simulink model "FullSystemSim_old"  (R2020a)
settings: Solver=VariableStepAuto  StartTime=0.0  StopTime=T_sim  RelTol=1e-3
values from neighbouring files (symbols this model uses):
  a_friction = 0    [FullSystem.m]
  b_friction = 1.19    [FullSystem.m]
  C_T_matrix = ex2(2:12,2:21)'    [FullSystem.m]
  J_wind = 5.245e-6 * 1000    (= 0.005245)    [FullSystem.m]
  K_t = 0.023    [FullSystem.m]    (also in WindTurbine.m = 82.8991502528)
  K_v = 0.023 / pi * 30    (= 0.219633821467)    [FullSystem.m]    (also in WindTurbine.m = 115.191730632)
  lambda_data_x = ex1(6, :)'    [FullSystem.m]
  lambda_opt = 2.1    [FullSystem.m]
  omega_0 = 100    [FullSystem.m]    (also in SystemControl_script.m = 100:)
  P_max_EL = 3    [FullSystem.m]
  P_max_FC = 1    [FullSystem.m]
  P_max_LED = 12*0.16*4    (= 7.68)    [FullSystem.m]
  P_max_SP = 0.5    [FullSystem.m]
  P_max_WT = 0.2    [FullSystem.m]
  R_LED_max = 75/4    (= 18.75)    [FullSystem.m]
  R_motor = 22.222    [FullSystem.m]
  R_turbine = 0.15    [FullSystem.m]    (also in SystemControl_script.m)
  r_wind_data_x = ex1(7, :)'    [FullSystem.m]
  rho_air = 1.225    [FullSystem.m]
  step_size = T_sim/n    (= 0.04)    [FullSystem.m]
  V_w_data_x = ex1(8,:)'    [FullSystem.m]
undefined symbols (not defined in the file or in its folder): DiscIntNeverNeededParam
libraries: fl_lib x37, nesl_utility x26, ee_lib x19, eePwmGenerator x4, simulink x2
settings Model: Creator=thequ  LastModifiedBy=fabia
settings DebuggingCC: ArithmeticOperatorsInVariantConditions=warning
settings SFSimCC: CustomCodeUndefinedFunction=UseInterfaceOnly

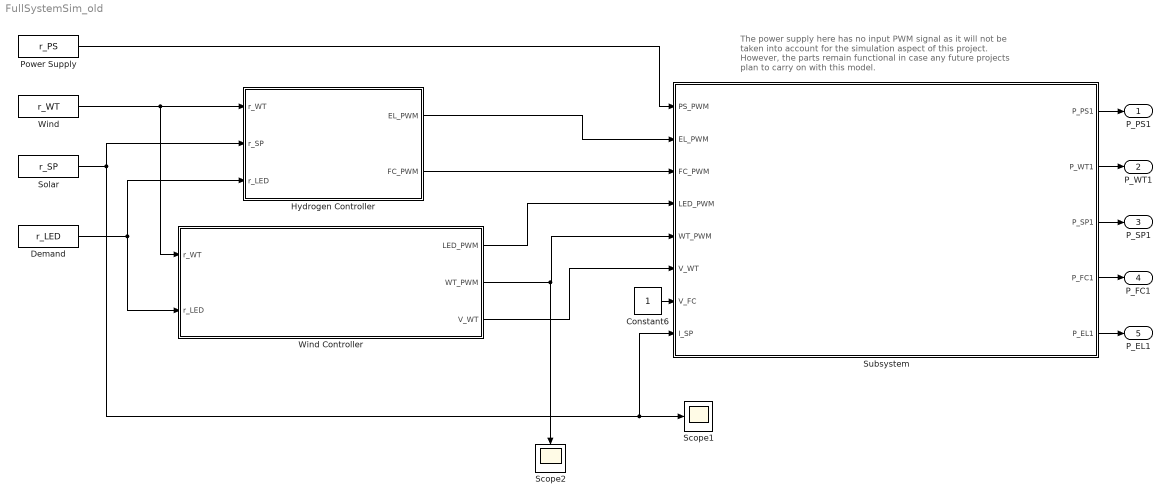
== system FullSystemSim_old ==
  note: The power supply here has no input PWM signal as it will not
      | be taken into account for the simulation aspect of this project.
      | However, the parts remain functional in case any future
      | projects plan to carry on with this model.
  Constant6 : Constant
  Demand : FromWorkspace  VariableName=r_LED  SampleTime=step_size  Interpolate=off  OutputAfterFinalValue=Holding final value
  Hydrogen Controller : Subsystem
  Power Supply : FromWorkspace  VariableName=r_PS  SampleTime=step_size  Interpolate=off  OutputAfterFinalValue=Holding final value
  Scope1 : Scope
  Scope2 : Scope
  Solar : FromWorkspace  VariableName=r_SP  SampleTime=step_size  Interpolate=off  OutputAfterFinalValue=Holding final value
  Subsystem : Subsystem
  Wind : FromWorkspace  VariableName=r_WT  SampleTime=step_size  Interpolate=off  OutputAfterFinalValue=Holding final value
  Wind Controller : Subsystem
  P_PS1 : Outport
  P_WT1 : Outport  Port=2
  P_SP1 : Outport  Port=3
  P_FC1 : Outport  Port=4
  P_EL1 : Outport  Port=5
  wires:
  Power Supply/1 -> Subsystem/1(PS_PWM)
  Subsystem/1(P_PS1) -> P_PS1/1
  Subsystem/2(P_WT1) -> P_WT1/1
  Subsystem/3(P_SP1) -> P_SP1/1
  Subsystem/4(P_FC1) -> P_FC1/1
  Subsystem/5(P_EL1) -> P_EL1/1
  Demand/1 -> Hydrogen Controller/3(r_LED), Wind Controller/2(r_LED)
  Wind Controller/3(V_WT) -> Subsystem/6(V_WT)
  Constant6/1 -> Subsystem/7(V_FC)
  Wind/1 -> Wind Controller/1(r_WT), Hydrogen Controller/1(r_WT)
  Solar/1 -> Hydrogen Controller/2(r_SP), Subsystem/8(I_SP), Scope1/1
  Wind Controller/2(WT_PWM) -> Subsystem/5(WT_PWM), Scope2/1
  Wind Controller/1(LED_PWM) -> Subsystem/4(LED_PWM)
  Hydrogen Controller/1(EL_PWM) -> Subsystem/2(EL_PWM)
  Hydrogen Controller/2(FC_PWM) -> Subsystem/3(FC_PWM)

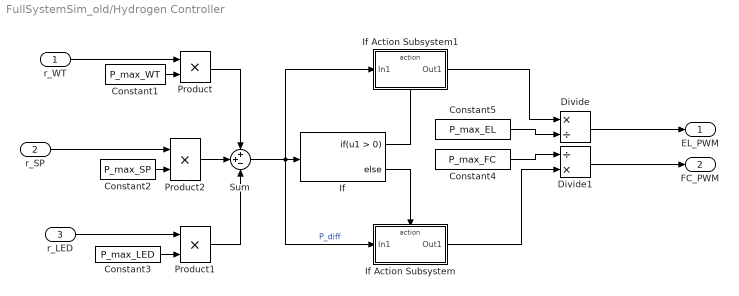
== system FullSystemSim_old/Hydrogen Controller ==
  r_WT : Inport
  r_SP : Inport  Port=2
  r_LED : Inport  Port=3
  Constant1 : Constant  Value=P_max_WT
  Constant2 : Constant  Value=P_max_SP
  Constant3 : Constant  Value=P_max_LED
  Constant4 : Constant  Value=P_max_FC
  Constant5 : Constant  Value=P_max_EL
  Divide : Product  Inputs=*/
  Divide1 : Product  Inputs=/*
  If : If
  If Action Subsystem : Subsystem  TreatAsAtomicUnit=on
  If Action Subsystem1 : Subsystem  TreatAsAtomicUnit=on
  Product : Product
  Product1 : Product
  Product2 : Product
  Sum : Sum  Inputs=++-
  EL_PWM : Outport
  FC_PWM : Outport  Port=2
  wires:
  Divide1/1 -> FC_PWM/1
  Product/1 -> Sum/1
  Divide/1 -> EL_PWM/1
  r_WT/1 -> Product/1
  If Action Subsystem/1(Out1) -> Divide1/2
  Constant5/1 -> Divide/2
  If/2 -> If Action Subsystem/Action
  Product1/1 -> Sum/3
  Sum/1 -> If Action Subsystem1/1(In1), If Action Subsystem/1(In1), If/1  "P_diff"
  Constant1/1 -> Product/2
  Constant4/1 -> Divide1/1
  If/1 -> If Action Subsystem1/Action
  If Action Subsystem1/1(Out1) -> Divide/1
  Constant3/1 -> Product1/2
  Constant2/1 -> Product2/2
  Product2/1 -> Sum/2
  r_LED/1 -> Product1/1
  r_SP/1 -> Product2/1

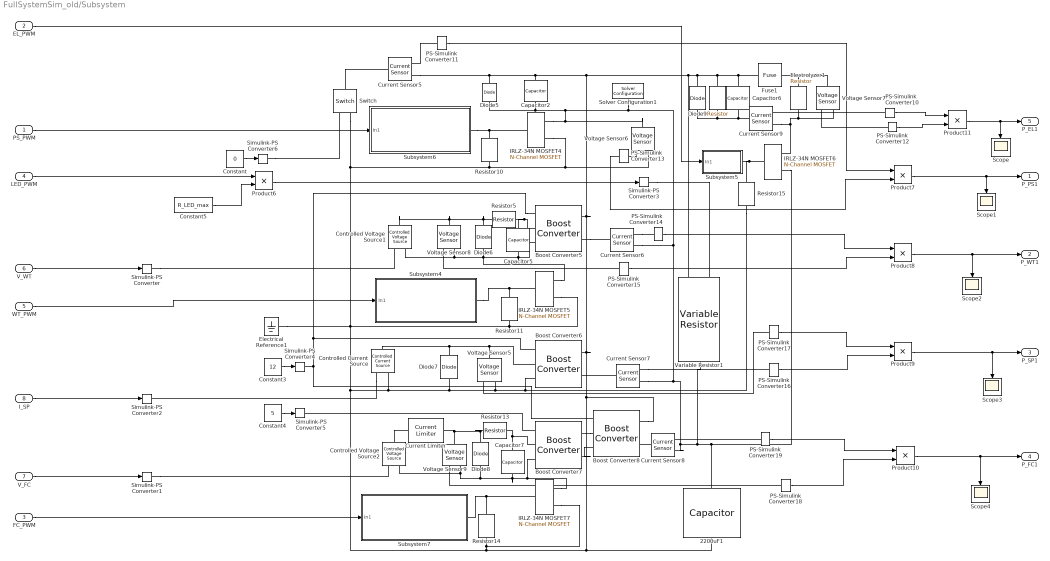
== system FullSystemSim_old/Subsystem ==
  PS_PWM : Inport
  EL_PWM : Inport  Port=2
  FC_PWM : Inport  Port=3
  LED_PWM : Inport  Port=4
  WT_PWM : Inport  Port=5
  V_WT : Inport  Port=6
  V_FC : Inport  Port=7
  I_SP : Inport  Port=8
  " " : fl_lib/Electrical/Electrical Elements/Resistor  R=16 Ohm  i_specify=off  i_priority=None  i=0 A  i_nominal_specify=off  i_nominal_unit=A  i_nominal_value=1  v_specify=off  v_priority=None  v=0 V  v_nominal_specify=off  v_nominal_unit=V  v_nominal_value=1
  2200uF1 : fl_lib/Electrical/Electrical Elements/Capacitor  c=2200 uF  r=0.014 Ohm  g=0 1/Ohm  i_specify=off  i_priority=None  i=0 A  i_nominal_specify=off  i_nominal_unit=A  i_nominal_value=1  v_specify=off  v_priority=None  v=0 V  v_nominal_specify=off  v_nominal_unit=V  v_nominal_value=1  vc_specify=off  vc_priority=High  vc=0 V  vc_nominal_specify=off  vc_nominal_unit=V  vc_nominal_value=1
  Boost Converter5 : ee_lib/Semiconductors & Converters/Converters/Boost Converter  device_type=4  Vf=0.8 V  Ron=0.001 Ohm  Rds=0.08 Ohm  Goff=1e-5 1/Ohm  Vth=2 V  Vgt=1 V  Vgt_off=-1 V  Ih=1 A  diode_param=2  diode_Vf=0.8 V  diode_Ron=0.001 Ohm  diode_Goff=1e-5 1/Ohm  diode_C=50 nF  diode_iRM=-235 A  diode_iF=300 A  diode_idot=-50 A/us  diode_trr_param=1  diode_trr_factor=3  diode_trr=15 us  diode_Qrr=1500 s*uA  Lf=1e-6 H  Cf=1e-7 F  Rf=1e-6 Ohm  snubber_type=0  Rs=0.1 Ohm  Cs=1e-7 F
      settings: SourceProductBaseCode=PS  InternalSimscapePortConfiguration="{\"Bottom\":[],\"Left\":[{\"id\":\"G\",\"label\":\"G\",\"type\":\"input\"},{\"id\":\"p1\",\"label\":\"1+\",\"type\":\"foundation.electrical.electrical\"},{\"id\":\"n1\",\"label\":\"1-\",\"type\":\"foundation.electrical.electrical\"}],\"Right\":[{\"id\":\"p2\",\"label\":\"2+\",\"type\":\"foundation.electrical.electrical\"},{\"id\":\"n2\",\"label\":\"2-\",\"type\":\"foundation.electrical.electrical\"}],\"Top\":[]}"
  Boost Converter6 : ee_lib/Semiconductors & Converters/Converters/Boost Converter  device_type=4  Vf=0.8 V  Ron=0.001 Ohm  Rds=0.08 Ohm  Goff=1e-5 1/Ohm  Vth=2 V  Vgt=1 V  Vgt_off=-1 V  Ih=1 A  diode_param=2  diode_Vf=0.8 V  diode_Ron=0.001 Ohm  diode_Goff=1e-5 1/Ohm  diode_C=50 nF  diode_iRM=-235 A  diode_iF=300 A  diode_idot=-50 A/us  diode_trr_param=1  diode_trr_factor=3  diode_trr=15 us  diode_Qrr=1500 s*uA  Lf=1e-6 H  Cf=1e-7 F  Rf=1e-6 Ohm  snubber_type=0  Rs=0.1 Ohm  Cs=1e-7 F
      settings: SourceProductBaseCode=PS  InternalSimscapePortConfiguration="{\"Bottom\":[],\"Left\":[{\"id\":\"G\",\"label\":\"G\",\"type\":\"input\"},{\"id\":\"p1\",\"label\":\"1+\",\"type\":\"foundation.electrical.electrical\"},{\"id\":\"n1\",\"label\":\"1-\",\"type\":\"foundation.electrical.electrical\"}],\"Right\":[{\"id\":\"p2\",\"label\":\"2+\",\"type\":\"foundation.electrical.electrical\"},{\"id\":\"n2\",\"label\":\"2-\",\"type\":\"foundation.electrical.electrical\"}],\"Top\":[]}"
  Boost Converter7 : ee_lib/Semiconductors & Converters/Converters/Boost Converter  device_type=4  Vf=0.8 V  Ron=0.001 Ohm  Rds=0.080 Ohm  Goff=1e-5 1/Ohm  Vth=0.9 V  Vgt=1 V  Vgt_off=-1 V  Ih=1 A  diode_param=2  diode_Vf=0.8 V  diode_Ron=0.001 Ohm  diode_Goff=1e-5 1/Ohm  diode_C=50 nF  diode_iRM=-235 A  diode_iF=300 A  diode_idot=-50 A/us  diode_trr_param=1  diode_trr_factor=3  diode_trr=15 us  diode_Qrr=1500 s*uA  Lf=1e-6 H  Cf=1e-7 F  Rf=1e-6 Ohm  snubber_type=0  Rs=0.1 Ohm  Cs=1e-7 F
      settings: SourceProductBaseCode=PS  InternalSimscapePortConfiguration="{\"Bottom\":[],\"Left\":[{\"id\":\"G\",\"label\":\"G\",\"type\":\"input\"},{\"id\":\"p1\",\"label\":\"1+\",\"type\":\"foundation.electrical.electrical\"},{\"id\":\"n1\",\"label\":\"1-\",\"type\":\"foundation.electrical.electrical\"}],\"Right\":[{\"id\":\"p2\",\"label\":\"2+\",\"type\":\"foundation.electrical.electrical\"},{\"id\":\"n2\",\"label\":\"2-\",\"type\":\"foundation.electrical.electrical\"}],\"Top\":[]}"
  Boost Converter8 : ee_lib/Semiconductors & Converters/Converters/Boost Converter  device_type=4  Vf=0.8 V  Ron=0.001 Ohm  Rds=0.08 Ohm  Goff=1e-5 1/Ohm  Vth=2 V  Vgt=1 V  Vgt_off=-1 V  Ih=1 A  diode_param=2  diode_Vf=0.8 V  diode_Ron=0.001 Ohm  diode_Goff=1e-5 1/Ohm  diode_C=50 nF  diode_iRM=-235 A  diode_iF=300 A  diode_idot=-50 A/us  diode_trr_param=1  diode_trr_factor=3  diode_trr=15 us  diode_Qrr=1500 s*uA  Lf=1e-6 H  Cf=1e-7 F  Rf=1e-6 Ohm  snubber_type=0  Rs=0.1 Ohm  Cs=1e-7 F
      settings: SourceProductBaseCode=PS  InternalSimscapePortConfiguration="{\"Bottom\":[],\"Left\":[{\"id\":\"G\",\"label\":\"G\",\"type\":\"input\"},{\"id\":\"p1\",\"label\":\"1+\",\"type\":\"foundation.electrical.electrical\"},{\"id\":\"n1\",\"label\":\"1-\",\"type\":\"foundation.electrical.electrical\"}],\"Right\":[{\"id\":\"p2\",\"label\":\"2+\",\"type\":\"foundation.electrical.electrical\"},{\"id\":\"n2\",\"label\":\"2-\",\"type\":\"foundation.electrical.electrical\"}],\"Top\":[]}"
  Capacitor2 : fl_lib/Electrical/Electrical Elements/Capacitor  c=1000 uF  r=0.02 Ohm  g=0 1/Ohm  i_specify=off  i_priority=None  i=0 A  i_nominal_specify=off  i_nominal_unit=A  i_nominal_value=1  v_specify=off  v_priority=None  v=0 V  v_nominal_specify=off  v_nominal_unit=V  v_nominal_value=1  vc_specify=off  vc_priority=High  vc=0 V  vc_nominal_specify=off  vc_nominal_unit=V  vc_nominal_value=1
  Capacitor5 : fl_lib/Electrical/Electrical Elements/Capacitor  c=1000 uF  r=0.02 Ohm  g=0 1/Ohm  i_specify=off  i_priority=None  i=0 A  i_nominal_specify=off  i_nominal_unit=A  i_nominal_value=1  v_specify=off  v_priority=None  v=0 V  v_nominal_specify=off  v_nominal_unit=V  v_nominal_value=1  vc_specify=off  vc_priority=High  vc=0 V  vc_nominal_specify=off  vc_nominal_unit=V  vc_nominal_value=1
  Capacitor6 : fl_lib/Electrical/Electrical Elements/Capacitor  c=1000 uF  r=0.20 Ohm  g=0 1/Ohm  i_specify=off  i_priority=None  i=0 A  i_nominal_specify=off  i_nominal_unit=A  i_nominal_value=1  v_specify=off  v_priority=None  v=0 V  v_nominal_specify=off  v_nominal_unit=V  v_nominal_value=1  vc_specify=off  vc_priority=High  vc=0 V  vc_nominal_specify=off  vc_nominal_unit=V  vc_nominal_value=1
  Capacitor7 : fl_lib/Electrical/Electrical Elements/Capacitor  c=1000 uF  r=0.02 Ohm  g=0 1/Ohm  i_specify=off  i_priority=None  i=0 A  i_nominal_specify=off  i_nominal_unit=A  i_nominal_value=1  v_specify=off  v_priority=None  v=0 V  v_nominal_specify=off  v_nominal_unit=V  v_nominal_value=1  vc_specify=off  vc_priority=High  vc=0 V  vc_nominal_specify=off  vc_nominal_unit=V  vc_nominal_value=1
  Constant : Constant  Value=0
  Constant3 : Constant  Value=12
  Constant4 : Constant  Value=5
  Constant5 : Constant  Value=R_LED_max
  Controlled Current Source : fl_lib/Electrical/Electrical Sources/Controlled Current Source
  Controlled Voltage Source1 : fl_lib/Electrical/Electrical Sources/Controlled Voltage Source
  Controlled Voltage Source2 : fl_lib/Electrical/Electrical Sources/Controlled Voltage Source
  Current Limiter : ee_lib/Semiconductors & Converters/Current Limiter  iLim=1.2 A  vLim=0.4 V  gLim=1e-3 1/Ohm  thermal_mass=100 J/K  initial_temperature=298.15 K
      settings: SourceProductBaseCode=PS  InternalSimscapePortConfiguration="{\"Bottom\":[],\"Left\":[{\"id\":\"p\",\"label\":\"+\",\"type\":\"foundation.electrical.electrical\"}],\"Right\":[{\"id\":\"n\",\"label\":\"-\",\"type\":\"foundation.electrical.electrical\"}],\"Top\":[]}"
  Current Sensor{5..9} (5 alike) : fl_lib/Electrical/Electrical Sensors/Current Sensor
  Diode5 : ee_lib/Semiconductors & Converters/Diode  ModelType=ee.enum.diode.modelType.pwl  Vf=0.6 V  Ron=0.3 Ohm  Goff=1e-8 S  prmExp=ee.enum.diode.expParam.useTwo  I12=[.0137, .545] A  V12=[.6, .7] V  IS=1e-12 A  ec=1  I1=0.0137 A  V1=0.6 V  RS=0 Ohm  Tmeas=25 degC  N_series=1  N_parallel=1  Rz=0.3 Ohm  BV=inf V  C_param=ee.enum.diode.capParam.fixed  CJ=5 pF  CJ0=5 pF  VJ=1 V  Mgrad=0.5  Vvec=[.1, 10, 100] V  Cvec=[3.5, 1, .4] pF  FC=0.5  Q_param=ee.enum.diode.recoveryParam.off  iRM=-7.15 A  iF=4 A  didt=-750 A/us  trr_factor=3  trr=115 ns  Qrr=1500 s*uA  TT=50 ns  tau=100 ns  T_param=ee.enum.diode.temperatureParam.off  IS_T2=1.25e-7 A  I1_T2=0.245 A  V1_T2=0.5 V  Tmeas2=125 degC  EG_param=ee.enum.diode.egapParam.material_si  EG=1.11 eV  XTI_param=ee.enum.diode.xtiParam.pn  XTI=3  dBVdT=0 V/K  Tdevice=25 degC  i_specify=off  i_priority=None  i=0 A  i_nominal_specify=off  i_nominal_unit=A  i_nominal_value=1  v_specify=off  v_priority=None  v=0 V  v_nominal_specify=off  v_nominal_unit=V  v_nominal_value=1  i_capacitor_specify=off  i_capacitor_priority=None  i_capacitor=0 A  i_capacitor_nominal_specify=off  i_capacitor_nominal_unit=A  i_capacitor_nominal_value=1  v_capacitor_specify=off  v_capacitor_priority=None  v_capacitor=0 V  v_capacitor_nominal_specify=off  v_capacitor_nominal_unit=V  v_capacitor_nominal_value=1  power_dissipated_specify=off  power_dissipated_priority=None  power_dissipated=0 W  power_dissipated_nominal_specify=off  power_dissipated_nominal_unit=W  power_dissipated_nominal_value=1  thermal_network_parameterization=ee.enum.thermalNetworkTopology.cauer  Rth=[0, 10] K/W  Rth_Foster=[4, 6] K/W  thermal_mass_parameterization=ee.enum.thermalNetwork.timeconstant  thermal_mass=[0, 1] J/K  thermal_mass_Foster=[1.5, 3] J/K  thermal_time_constant=[0, 10] s  thermal_time_constant_Foster=[6, 18] s  thermal_mass_initial_temperatures=[25, 25] degC
  Diode6 : ee_lib/Semiconductors & Converters/Diode  ModelType=ee.enum.diode.modelType.pwl  Vf=0.85 V  Ron=0.05 Ohm  Goff=1e-8 S  prmExp=ee.enum.diode.expParam.useTwo  I12=[.0137, .545] A  V12=[.6, .7] V  IS=1e-12 A  ec=1  I1=0.0137 A  V1=0.6 V  RS=0 Ohm  Tmeas=25 degC  N_series=1  N_parallel=1  Rz=0.3 Ohm  BV=inf V  C_param=ee.enum.diode.capParam.fixed  CJ=5 pF  CJ0=5 pF  VJ=1 V  Mgrad=0.5  Vvec=[.1, 10, 100] V  Cvec=[3.5, 1, .4] pF  FC=0.5  Q_param=ee.enum.diode.recoveryParam.off  iRM=-7.15 A  iF=4 A  didt=-750 A/us  trr_factor=3  trr=115 ns  Qrr=1500 s*uA  TT=50 ns  tau=100 ns  T_param=ee.enum.diode.temperatureParam.off  IS_T2=1.25e-7 A  I1_T2=0.245 A  V1_T2=0.5 V  Tmeas2=125 degC  EG_param=ee.enum.diode.egapParam.material_si  EG=1.11 eV  XTI_param=ee.enum.diode.xtiParam.pn  XTI=3  dBVdT=0 V/K  Tdevice=25 degC  i_specify=off  i_priority=None  i=0 A  i_nominal_specify=off  i_nominal_unit=A  i_nominal_value=1  v_specify=off  v_priority=None  v=0 V  v_nominal_specify=off  v_nominal_unit=V  v_nominal_value=1  i_capacitor_specify=off  i_capacitor_priority=None  i_capacitor=0 A  i_capacitor_nominal_specify=off  i_capacitor_nominal_unit=A  i_capacitor_nominal_value=1  v_capacitor_specify=off  v_capacitor_priority=None  v_capacitor=0 V  v_capacitor_nominal_specify=off  v_capacitor_nominal_unit=V  v_capacitor_nominal_value=1  power_dissipated_specify=off  power_dissipated_priority=None  power_dissipated=0 W  power_dissipated_nominal_specify=off  power_dissipated_nominal_unit=W  power_dissipated_nominal_value=1  thermal_network_parameterization=ee.enum.thermalNetworkTopology.cauer  Rth=[0, 10] K/W  Rth_Foster=[4, 6] K/W  thermal_mass_parameterization=ee.enum.thermalNetwork.timeconstant  thermal_mass=[0, 1] J/K  thermal_mass_Foster=[1.5, 3] J/K  thermal_time_constant=[0, 10] s  thermal_time_constant_Foster=[6, 18] s  thermal_mass_initial_temperatures=[25, 25] degC
  Diode7 : ee_lib/Semiconductors & Converters/Diode  ModelType=ee.enum.diode.modelType.pwl  Vf=0.85 V  Ron=0.05 Ohm  Goff=1e-8 S  prmExp=ee.enum.diode.expParam.useTwo  I12=[.0137, .545] A  V12=[.6, .7] V  IS=1e-12 A  ec=1  I1=0.0137 A  V1=0.6 V  RS=0 Ohm  Tmeas=25 degC  N_series=1  N_parallel=1  Rz=0.3 Ohm  BV=inf V  C_param=ee.enum.diode.capParam.fixed  CJ=5 pF  CJ0=5 pF  VJ=1 V  Mgrad=0.5  Vvec=[.1, 10, 100] V  Cvec=[3.5, 1, .4] pF  FC=0.5  Q_param=ee.enum.diode.recoveryParam.off  iRM=-7.15 A  iF=4 A  didt=-750 A/us  trr_factor=3  trr=115 ns  Qrr=1500 s*uA  TT=50 ns  tau=100 ns  T_param=ee.enum.diode.temperatureParam.off  IS_T2=1.25e-7 A  I1_T2=0.245 A  V1_T2=0.5 V  Tmeas2=125 degC  EG_param=ee.enum.diode.egapParam.material_si  EG=1.11 eV  XTI_param=ee.enum.diode.xtiParam.pn  XTI=3  dBVdT=0 V/K  Tdevice=25 degC  i_specify=off  i_priority=None  i=0 A  i_nominal_specify=off  i_nominal_unit=A  i_nominal_value=1  v_specify=off  v_priority=None  v=0 V  v_nominal_specify=off  v_nominal_unit=V  v_nominal_value=1  i_capacitor_specify=off  i_capacitor_priority=None  i_capacitor=0 A  i_capacitor_nominal_specify=off  i_capacitor_nominal_unit=A  i_capacitor_nominal_value=1  v_capacitor_specify=off  v_capacitor_priority=None  v_capacitor=0 V  v_capacitor_nominal_specify=off  v_capacitor_nominal_unit=V  v_capacitor_nominal_value=1  power_dissipated_specify=off  power_dissipated_priority=None  power_dissipated=0 W  power_dissipated_nominal_specify=off  power_dissipated_nominal_unit=W  power_dissipated_nominal_value=1  thermal_network_parameterization=ee.enum.thermalNetworkTopology.cauer  Rth=[0, 10] K/W  Rth_Foster=[4, 6] K/W  thermal_mass_parameterization=ee.enum.thermalNetwork.timeconstant  thermal_mass=[0, 1] J/K  thermal_mass_Foster=[1.5, 3] J/K  thermal_time_constant=[0, 10] s  thermal_time_constant_Foster=[6, 18] s  thermal_mass_initial_temperatures=[25, 25] degC
  Diode8 : ee_lib/Semiconductors & Converters/Diode  ModelType=ee.enum.diode.modelType.pwl  Vf=0.85 V  Ron=0.05 Ohm  Goff=1e-8 S  prmExp=ee.enum.diode.expParam.useTwo  I12=[.0137, .545] A  V12=[.6, .7] V  IS=1e-12 A  ec=1  I1=0.0137 A  V1=0.6 V  RS=0 Ohm  Tmeas=25 degC  N_series=1  N_parallel=1  Rz=0.3 Ohm  BV=inf V  C_param=ee.enum.diode.capParam.fixed  CJ=5 pF  CJ0=5 pF  VJ=1 V  Mgrad=0.5  Vvec=[.1, 10, 100] V  Cvec=[3.5, 1, .4] pF  FC=0.5  Q_param=ee.enum.diode.recoveryParam.off  iRM=-7.15 A  iF=4 A  didt=-750 A/us  trr_factor=3  trr=115 ns  Qrr=1500 s*uA  TT=50 ns  tau=100 ns  T_param=ee.enum.diode.temperatureParam.off  IS_T2=1.25e-7 A  I1_T2=0.245 A  V1_T2=0.5 V  Tmeas2=125 degC  EG_param=ee.enum.diode.egapParam.material_si  EG=1.11 eV  XTI_param=ee.enum.diode.xtiParam.pn  XTI=3  dBVdT=0 V/K  Tdevice=25 degC  i_specify=off  i_priority=None  i=0 A  i_nominal_specify=off  i_nominal_unit=A  i_nominal_value=1  v_specify=off  v_priority=None  v=0 V  v_nominal_specify=off  v_nominal_unit=V  v_nominal_value=1  i_capacitor_specify=off  i_capacitor_priority=None  i_capacitor=0 A  i_capacitor_nominal_specify=off  i_capacitor_nominal_unit=A  i_capacitor_nominal_value=1  v_capacitor_specify=off  v_capacitor_priority=None  v_capacitor=0 V  v_capacitor_nominal_specify=off  v_capacitor_nominal_unit=V  v_capacitor_nominal_value=1  power_dissipated_specify=off  power_dissipated_priority=None  power_dissipated=0 W  power_dissipated_nominal_specify=off  power_dissipated_nominal_unit=W  power_dissipated_nominal_value=1  thermal_network_parameterization=ee.enum.thermalNetworkTopology.cauer  Rth=[0, 10] K/W  Rth_Foster=[4, 6] K/W  thermal_mass_parameterization=ee.enum.thermalNetwork.timeconstant  thermal_mass=[0, 1] J/K  thermal_mass_Foster=[1.5, 3] J/K  thermal_time_constant=[0, 10] s  thermal_time_constant_Foster=[6, 18] s  thermal_mass_initial_temperatures=[25, 25] degC
  Diode9 : ee_lib/Semiconductors & Converters/Diode  ModelType=ee.enum.diode.modelType.pwl  Vf=0.7 V  Ron=0.3 Ohm  Goff=1e-8 S  prmExp=ee.enum.diode.expParam.useTwo  I12=[.0137, .545] A  V12=[.6, .7] V  IS=1e-12 A  ec=1  I1=0.0137 A  V1=0.6 V  RS=0 Ohm  Tmeas=25 degC  N_series=1  N_parallel=1  Rz=0.3 Ohm  BV=inf V  C_param=ee.enum.diode.capParam.fixed  CJ=5 pF  CJ0=5 pF  VJ=1 V  Mgrad=0.5  Vvec=[.1, 10, 100] V  Cvec=[3.5, 1, .4] pF  FC=0.5  Q_param=ee.enum.diode.recoveryParam.off  iRM=-7.15 A  iF=4 A  didt=-750 A/us  trr_factor=3  trr=115 ns  Qrr=1500 s*uA  TT=50 ns  tau=100 ns  T_param=ee.enum.diode.temperatureParam.off  IS_T2=1.25e-7 A  I1_T2=0.245 A  V1_T2=0.5 V  Tmeas2=125 degC  EG_param=ee.enum.diode.egapParam.material_si  EG=1.11 eV  XTI_param=ee.enum.diode.xtiParam.pn  XTI=3  dBVdT=0 V/K  Tdevice=25 degC  i_specify=off  i_priority=None  i=0 A  i_nominal_specify=off  i_nominal_unit=A  i_nominal_value=1  v_specify=off  v_priority=None  v=0 V  v_nominal_specify=off  v_nominal_unit=V  v_nominal_value=1  i_capacitor_specify=off  i_capacitor_priority=None  i_capacitor=0 A  i_capacitor_nominal_specify=off  i_capacitor_nominal_unit=A  i_capacitor_nominal_value=1  v_capacitor_specify=off  v_capacitor_priority=None  v_capacitor=0 V  v_capacitor_nominal_specify=off  v_capacitor_nominal_unit=V  v_capacitor_nominal_value=1  power_dissipated_specify=off  power_dissipated_priority=None  power_dissipated=0 W  power_dissipated_nominal_specify=off  power_dissipated_nominal_unit=W  power_dissipated_nominal_value=1  thermal_network_parameterization=ee.enum.thermalNetworkTopology.cauer  Rth=[0, 10] K/W  Rth_Foster=[4, 6] K/W  thermal_mass_parameterization=ee.enum.thermalNetwork.timeconstant  thermal_mass=[0, 1] J/K  thermal_mass_Foster=[1.5, 3] J/K  thermal_time_constant=[0, 10] s  thermal_time_constant_Foster=[6, 18] s  thermal_mass_initial_temperatures=[25, 25] degC
  Electrical Reference1 : fl_lib/Electrical/Electrical Elements/Electrical Reference
  Electrolyzer1 : fl_lib/Electrical/Electrical Elements/Resistor  R=4 Ohm  i_specify=off  i_priority=None  i=0 A  i_nominal_specify=off  i_nominal_unit=A  i_nominal_value=1  v_specify=off  v_priority=None  v=0 V  v_nominal_specify=off  v_nominal_unit=V  v_nominal_value=1
  Fuse1 : ee_lib/Switches & Breakers/Fuse  prm=1  I_rated=1.5 A  melt_margin=1  T_fuse=0 s  I2t=1 s*A^2  I_vec=[1.9, 2, 2.5, 30] A  t_vec=[10000, 1, .3, .001] s  R_closed=0.01 Ohm  G_open=1e-8 1/Ohm  exposemeasurement=ee.enum.exposemeasurement.hidden
      settings: SourceProductBaseCode=PS  InternalSimscapePortConfiguration="{\"Bottom\":[],\"Left\":[{\"id\":\"p\",\"label\":\"\",\"type\":\"foundation.electrical.electrical\"}],\"Right\":[{\"id\":\"n\",\"label\":\"\",\"type\":\"foundation.electrical.electrical\"}],\"Top\":[]}"
  IRLZ-34N MOSFET{4..7} (4 alike) : ee_lib/Semiconductors & Converters/N-Channel MOSFET  paramTerminal=ee.enum.mosfet.numberOfTerminals.three  parameterization=1  prmDatasheet=1  prmEquCoeff=1  Beta=5.0 A/V^2  Rds=0.046 Ohm  Id=30 A  Vgs=5 V  Vth=1.5 V  Vth0=1.7 V  lam=0 1/V  gamma_vth=0.5 V^0.50000  phib=0.5 V  Vth1=1.9071 V  Vbs1=-1 V  Vth2=2.066 V  Vbs2=-2 V  Tmeas=25 degC  RS=0.0001 Ohm  RD=0.01 Ohm  RB=0.001 Ohm  C_param=1  C_GS=270 pF  C_GD=80 pF  C_DS=0 pF  C_iss=350 pF  C_rss=80 pF  C_oss=0 pF  charge_linearity_param=1  C_OX=200 pF  V_C_OX=-0.5 V  C_iss_vec=[720, 700, 590, 470, 390, 310] pF  C_rss_vec=[450, 400, 300, 190, 95, 55] pF  C_oss_vec=[900, 810, 690, 420, 270, 170] pF  C_GS_vec=[270, 300, 290, 280, 295, 255] pF  C_GD_vec=[450, 400, 300, 190, 95, 55] pF  C_DS_vec=[450, 410, 390, 230, 175, 115] pF  C_Vds_vec=[.1, .3, 1, 3, 10, 30] V  V_GS_for_cap_data=0 V  charge_linearity_param_vgb=ee.enum.mosfet.cgbLinearity.instantly  IsDiode=0 A  Vbi=0.6 V  n=1  Cj0Diode=0 pF  TT=50e-9 s  dVth_dT=-6 mV/K  dVth0_dT=-6 mV/K  Rds_T2=0.037 Ohm  Tmeas2=125 degC  BEXDatasheet=-1.5  BEXEquCoeff=-1.5  etaisDatasheet=3  etaisEquCoeff=3  TdeviceDatasheet=25 degC  TdeviceEquCoeff=25 degC  thermal_network_parameterization=ee.enum.thermalNetworkTopology.cauer  Rth=[0, 10] K/W  Rth_Foster=[4, 6] K/W  thermal_mass_parameterization=ee.enum.thermalNetwork.timeconstant  thermal_mass=[0, 1] J/K  thermal_mass_Foster=[1.5, 3] J/K  thermal_time_constant=[0, 10] s  thermal_time_constant_Foster=[6, 18] s  thermal_mass_initial_temperatures=[25, 25] degC  betaref=18 A/V^2  Vfbref=-1.1 V  gamma=3.5 V^0.50000  phib2ref=1 V  thesatref=0.4 1/V  alpha=0  Vp=5e-2 V  thesrref=0 1/V  m=8  Tref=25 degC  Cox=1500 pF  Cgso=100 pF  Cgdo=14 pF  Rsref=2e-3 Ohm  Rdref=0.17 Ohm  Rgref=8.4 Ohm  Rbref=2e-3 Ohm  Isref=5.2e-13 A  Cj0=480 pF  Tprm=1  etabet=1.3  Stvfb=5e-4 V/K  Stphib=-8.5e-4 V/K  etasat=1.04  etasr=0.65  etar=0.95  etais=3  Tsim=25 degC  T0=[25, 25] degC
  PS-Simulink Converter{10..19} (10 alike) : nesl_utility/PS-Simulink Converter  PhysicalDomain=network_engine_domain  SubClassName=ps_output  LeftPortType=input  RightPortType=output  PseudoPeriodic=off  Frequencies=[]  Unit=inherit  AffineConversion=off
  Product{6..11} (6 alike) : Product
  Resistor{10..11,14..15} (4 alike) : fl_lib/Electrical/Electrical Elements/Resistor  R=10000 Ohm  i_specify=off  i_priority=None  i=0 A  i_nominal_specify=off  i_nominal_unit=A  i_nominal_value=1  v_specify=off  v_priority=None  v=0 V  v_nominal_specify=off  v_nominal_unit=V  v_nominal_value=1
  Resistor13 : fl_lib/Electrical/Electrical Elements/Resistor  R=16 Ohm  i_specify=off  i_priority=None  i=0 A  i_nominal_specify=off  i_nominal_unit=A  i_nominal_value=1  v_specify=off  v_priority=None  v=0 V  v_nominal_specify=off  v_nominal_unit=V  v_nominal_value=1
  Resistor5 : fl_lib/Electrical/Electrical Elements/Resistor  R=16 Ohm  i_specify=off  i_priority=None  i=0 A  i_nominal_specify=off  i_nominal_unit=A  i_nominal_value=1  v_specify=off  v_priority=None  v=0 V  v_nominal_specify=off  v_nominal_unit=V  v_nominal_value=1
  Scope{,1..4} (5 alike) : Scope
  Simulink-PS Converter : nesl_utility/Simulink-PS Converter  PhysicalDomain=network_engine_domain  SubClassName=ps_input  LeftPortType=input  RightPortType=output  PseudoPeriodic=off  Frequencies=[]  NoiseDistribution=none  NoiseParameters=[]  Unit=1  AffineConversion=off  FilteringAndDerivatives=filter  SimscapeFilterOrder=1  InputFilterTimeConstant=0.001  UdotUserProvided=0
  Simulink-PS Converter{1..6} (6 alike) : nesl_utility/Simulink-PS Converter  PhysicalDomain=network_engine_domain  SubClassName=ps_input  LeftPortType=input  RightPortType=output  PseudoPeriodic=off  Frequencies=[]  NoiseDistribution=none  NoiseParameters=[]  Unit=1  AffineConversion=off  FilteringAndDerivatives=provide  SimscapeFilterOrder=1  InputFilterTimeConstant=0.001  UdotUserProvided=0
  Solver Configuration1 : nesl_utility/Solver Configuration  PhysicalDomain=network_engine_domain  SubClassName=solver  LeftPortType=input  RightPortType=generic  Tones=[]  Harmonics=[]  SimulateNoise=off  Profile=off  UseLocalSampling=off  EnableSwitchedLinearOptims=on  FrequencyDomain=off  UseCCode=off  RelTol=0.001  AbsTol=1e-06  MinStep=1e-09  ToWorkspace=off  RevertToSquareIcSolve=off  NumHomotopyIterations=100  PhasorMode=off  PhasorModeNumHarmonics=1  DoDC=off  ResidualTolerance=1e-09  UseLocalSolver=off  LocalSolverChoice=NE_BACKWARD_EULER_ADVANCER  LocalSolverSampleTime=0.001  DoFixedCost=off  MaxNonlinIter=3  MaxModeIter=2  LinearAlgebra=auto  EquationFormulation=NE_TIME_EF  DelaysMemoryBudget=1024  AutomaticFiltering=on  FilteringTimeConstant=0.001  PartitionStorageMethod=AS_NEEDED  PartitionMemoryBudget=1024  PartitionMethod=ROBUST
  Subsystem4 : Subsystem
  Subsystem5 : Subsystem
  Subsystem6 : Subsystem
  Subsystem7 : Subsystem
  Switch : fl_lib/Electrical/Electrical Elements/Switch  R_closed=0.01 Ohm  G_open=1e-8 1/Ohm  Threshold=0.5  i_specify=off  i_priority=None  i=0 A  i_nominal_specify=off  i_nominal_unit=A  i_nominal_value=1  v_specify=off  v_priority=None  v=0 V  v_nominal_specify=off  v_nominal_unit=V  v_nominal_value=1
  Variable Resistor1 : fl_lib/Electrical/Electrical Elements/Variable Resistor  Rmin=25 Ohm  i_specify=off  i_priority=None  i=0 A  i_nominal_specify=off  i_nominal_unit=A  i_nominal_value=1  v_specify=off  v_priority=None  v=0 V  v_nominal_specify=off  v_nominal_unit=V  v_nominal_value=1
  Voltage Sensor{5..9} (5 alike) : fl_lib/Electrical/Electrical Sensors/Voltage Sensor
  P_PS1 : Outport
  P_WT1 : Outport  Port=2
  P_SP1 : Outport  Port=3
  P_FC1 : Outport  Port=4
  P_EL1 : Outport  Port=5
  wires:
  PS-Simulink Converter14/1 -> Product8/1
  FC_PWM/1 -> Subsystem7/1(In1)
  EL_PWM/1 -> Subsystem5/1(In1)
  Constant3/1 -> Simulink-PS Converter4/1
  PS-Simulink Converter17/1 -> Product9/1
  Product6/1 -> Simulink-PS Converter3/1
  PS-Simulink Converter13/1 -> Product7/2
  PS-Simulink Converter15/1 -> Product8/2
  WT_PWM/1 -> Subsystem4/1(In1)
  PS-Simulink Converter12/1 -> Product11/2
  Constant5/1 -> Product6/2
  PS-Simulink Converter11/1 -> Product7/1
  Constant4/1 -> Simulink-PS Converter5/1
  PS-Simulink Converter18/1 -> Product10/2
  PS-Simulink Converter16/1 -> Product9/2
  PS-Simulink Converter10/1 -> Product11/1
  PS-Simulink Converter19/1 -> Product10/1
  PS_PWM/1 -> Subsystem6/1(In1)
  LED_PWM/1 -> Product6/1
  V_WT/1 -> Simulink-PS Converter/1
  V_FC/1 -> Simulink-PS Converter1/1
  I_SP/1 -> Simulink-PS Converter2/1
  Product11/1 -> Scope/1, P_EL1/1
  Product7/1 -> Scope1/1, P_PS1/1
  Product8/1 -> Scope2/1, P_WT1/1
  Product9/1 -> P_SP1/1, Scope3/1
  Product10/1 -> Scope4/1, P_FC1/1
  Constant/1 -> Simulink-PS Converter6/1
  connections:
  Boost Converter7/RConn1 -- Boost Converter8/LConn2
  Voltage Sensor9/RConn2 -- Controlled Voltage Source2/RConn2 -- Boost Converter7/LConn3 -- IRLZ-34N MOSFET7/RConn1 -- Capacitor7/RConn1 -- Diode8/LConn1
  Current Sensor7/RConn2 -- Solver Configuration1/RConn1 -- Capacitor2/RConn1 -- Diode5/LConn1 -- IRLZ-34N MOSFET4/RConn1 -- Voltage Sensor6/LConn1 -- Current Sensor6/RConn2 -- Current Sensor8/RConn2 -- IRLZ-34N MOSFET6/RConn2 -- 2200uF1/LConn1 -- Variable Resistor1/RConn1
  Diode6/RConn1 -- Controlled Voltage Source1/LConn1 -- Voltage Sensor8/LConn1 -- Resistor5/LConn1
  Controlled Voltage Source2/LConn1 -- Current Limiter/LConn1
  Boost Converter5/LConn2 -- Resistor5/RConn1 -- Capacitor5/LConn1
  Simulink-PS Converter3/RConn1 -- Variable Resistor1/LConn1
  Electrolyzer1/LConn1 -- Fuse1/RConn1 -- Voltage Sensor7/LConn1
  Subsystem5/RConn1 -- IRLZ-34N MOSFET6/LConn1 -- Resistor15/LConn1
  Boost Converter7/LConn1 -- Simulink-PS Converter5/RConn1
  Boost Converter5/LConn1 -- Simulink-PS Converter4/RConn1 -- Boost Converter8/LConn1 -- Boost Converter6/LConn1
  PS-Simulink Converter15/LConn1 -- Voltage Sensor8/RConn1
  Current Sensor9/RConn2 -- Electrolyzer1/RConn1 -- Voltage Sensor7/RConn2 -- IRLZ-34N MOSFET6/RConn1
  Current Sensor8/LConn1 -- Boost Converter8/RConn2
  " "/LConn1 -- Capacitor6/LConn1 -- Fuse1/LConn1 -- Diode9/RConn1 -- Current Sensor5/RConn2 -- Diode5/RConn1 -- Capacitor2/LConn1 -- 2200uF1/RConn1 -- IRLZ-34N MOSFET7/RConn2 -- Resistor14/RConn1 -- Electrical Reference1/LConn1 -- Switch/RConn2 -- Resistor10/RConn1 -- Voltage Sensor6/RConn2 -- IRLZ-34N MOSFET4/RConn2 -- IRLZ-34N MOSFET5/RConn2 -- Resistor11/RConn1 -- Voltage Sensor5/RConn2 -- Resistor15/RConn1 -- Boost Converter6/LConn3 -- Diode7/LConn1 -- Controlled Current Source/RConn2 -- Boost Converter8/RConn1 -- Boost Converter6/RConn1 -- Boost Converter5/RConn1 -- Variable Resistor1/LConn2
  Resistor10/LConn1 -- IRLZ-34N MOSFET4/LConn1 -- Subsystem6/RConn1
  Resistor11/LConn1 -- IRLZ-34N MOSFET5/LConn1 -- Subsystem4/RConn1
  Capacitor6/RConn1 -- " "/RConn1 -- Diode9/LConn1 -- Current Sensor9/LConn1
  Current Sensor6/RConn1 -- PS-Simulink Converter14/LConn1
  Subsystem7/RConn1 -- Resistor14/LConn1 -- IRLZ-34N MOSFET7/LConn1
  Boost Converter5/LConn3 -- IRLZ-34N MOSFET5/RConn1 -- Controlled Voltage Source1/RConn2 -- Voltage Sensor8/RConn2 -- Diode6/LConn1 -- Capacitor5/RConn1
  Capacitor7/LConn1 -- Boost Converter7/LConn2 -- Resistor13/RConn1
  Boost Converter6/LConn2 -- Controlled Current Source/LConn1 -- Diode7/RConn1 -- Voltage Sensor5/LConn1
  Current Sensor5/LConn1 -- Switch/LConn1
  Current Sensor7/RConn1 -- PS-Simulink Converter16/LConn1
  PS-Simulink Converter12/LConn1 -- Voltage Sensor7/RConn1
  PS-Simulink Converter18/LConn1 -- Voltage Sensor9/RConn1
  PS-Simulink Converter10/LConn1 -- Current Sensor9/RConn1
  PS-Simulink Converter19/LConn1 -- Current Sensor8/RConn1
  PS-Simulink Converter17/LConn1 -- Voltage Sensor5/RConn1
  PS-Simulink Converter11/LConn1 -- Current Sensor5/RConn1
  Boost Converter7/RConn2 -- Boost Converter8/LConn3
  Boost Converter5/RConn2 -- Current Sensor6/LConn1
  PS-Simulink Converter13/LConn1 -- Voltage Sensor6/RConn1
  Current Sensor7/LConn1 -- Boost Converter6/RConn2
  Voltage Sensor9/LConn1 -- Current Limiter/RConn1 -- Resistor13/LConn1 -- Diode8/RConn1
  Simulink-PS Converter/RConn1 -- Controlled Voltage Source1/RConn1
  Simulink-PS Converter1/RConn1 -- Controlled Voltage Source2/RConn1
  Controlled Current Source/RConn1 -- Simulink-PS Converter2/RConn1
  Simulink-PS Converter6/RConn1 -- Switch/RConn1

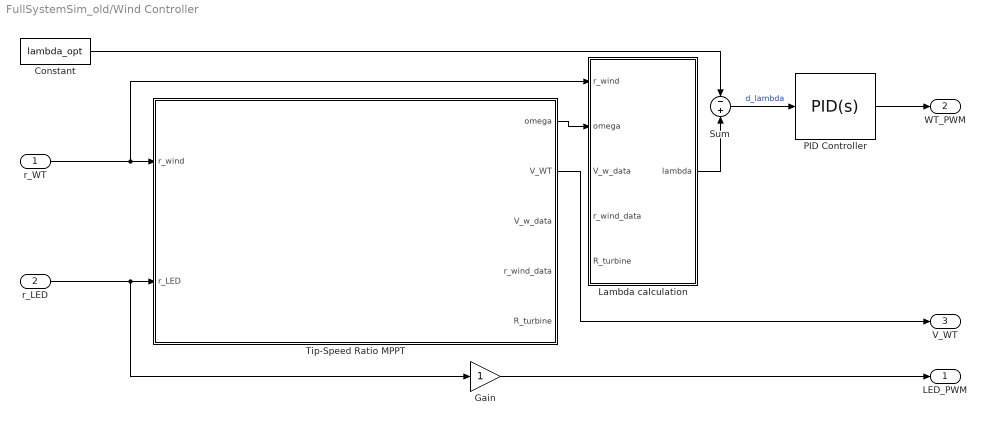
== system FullSystemSim_old/Wind Controller ==
  r_WT : Inport
  r_LED : Inport  Port=2
  Constant : Constant  Value=lambda_opt
  Gain : Gain
  Lambda calculation : Subsystem
  PID Controller : simulink/Continuous/PID Controller  Controller=PID  Form=Parallel  TimeDomain=Continuous-time  UseExternalTs=off  SampleTime=-1  IntegratorMethod=Forward Euler  FilterMethod=Forward Euler  ControllerParametersSource=internal  P=1  I=1  D=0  UseFilter=on  N=100  TunerSelectOption=Transfer Function Based (PID Tuner App)  InitialConditionSource=internal  InitialConditionForIntegrator=0  InitialConditionForFilter=0  DifferentiatorICPrevScaledInput=0  ExternalReset=none  TrackingMode=off  Kt=1  LimitOutput=off  UpperSaturationLimit=inf  LowerSaturationLimit=-inf  LinearizeAsGain=on  AntiWindupMode=none  Kb=1  POutMin=[]  POutMax=[]  IOutMin=[]  IOutMax=[]  DOutMin=[]  DOutMax=[]  NOutMin=[]  NOutMax=[]  SumOutMin=[]  SumOutMax=[]  SaturationOutMin=[]  SaturationOutMax=[]  PParamMin=[]  PParamMax=[]  IParamMin=[]  IParamMax=[]  DParamMin=[]  DParamMax=[]  NParamMin=[]  NParamMax=[]  KbParamMin=[]  KbParamMax=[]  KtParamMin=[]  KtParamMax=[]  KbOutMin=[]  KbOutMax=[]  KtOutMin=[]  KtOutMax=[]  IntegratorOutMin=[]  IntegratorOutMax=[]  FilterOutMin=[]  FilterOutMax=[]  SumI1OutMin=[]  SumI1OutMax=[]  SumI2OutMin=[]  SumI2OutMax=[]  SumI3OutMin=[]  SumI3OutMax=[]  SumI4OutMin=[]  SumI4OutMax=[]  SumDOutMin=[]  SumDOutMax=[]  DifferentiatorOutMin=[]  DifferentiatorOutMax=[]  FilterDiffOutCoefMin=[]  FilterDiffOutCoefMax=[]  ReciprocalOutMin=[]  ReciprocalOutMax=[]  SumDenOutMin=[]  SumDenOutMax=[]  SumNumOutMin=[]  SumNumOutMax=[]  DivideOutMin=[]  DivideOutMax=[]  UdiffTsProdOutMin=[]  UdiffTsProdOutMax=[]  NTsProdOutMin=[]  NTsProdOutMax=[]  UintegralTsProdOutMin=[]  UintegralTsProdOutMax=[]  UngainTsProdOutMin=[]  UngainTsProdOutMax=[]  IntegratorContinuousStateAttributes=''  IntegratorStateMustResolveToSignalObject=off  IntegratorRTWStateStorageClass=Auto  FilterContinuousStateAttributes=''  FilterStateMustResolveToSignalObject=off  FilterRTWStateStorageClass=Auto  ParallelPVariant=InternalParameters  IdealPVariant=Disabled  IVariant=InternalParameters  DVariant=InternalParameters  IntegratorVariant=Continuous  SatVariant=Disabled  AWVariant=Passthrough  PCopyVariant=Disabled  TRVariant=Disabled  FdbkBlocksVariant=Forward  IdealPFdbkVariant=Disabled  SatFdbkVariant=Disabled  DerivativeFilterVariant=ContFilter  NVariant=InternalParameters  NCopyVariant=Disabled  FilterICVariant=InternalICsFilter  IntegratorICVariant=InternalICs  ExternalResetVariant=Disabled  TRSumVariant=Passthrough  SumFdbkVariant=Disabled  SumVariant=Sum_PID  TsampFilterVariant=InternalTs  TsampNgainVariant=Passthrough  TsampIntegralVariant=Passthrough
  Sum : Sum  Inputs=-+
  Tip-Speed Ratio MPPT : Subsystem
  LED_PWM : Outport
  WT_PWM : Outport  Port=2
  V_WT : Outport  Port=3
  wires:
  Sum/1 -> PID Controller/1  "d_lambda"
  ? -> Lambda calculation/5(R_turbine)
  r_LED/1 -> Gain/1, Tip-Speed Ratio MPPT/2(r_LED)
  ? -> Lambda calculation/4(r_wind_data)
  ? -> Lambda calculation/3(V_w_data)
  Tip-Speed Ratio MPPT/1(omega) -> Lambda calculation/2(omega)
  r_WT/1 -> Lambda calculation/1(r_wind), Tip-Speed Ratio MPPT/1(r_wind)
  Constant/1 -> Sum/1
  PID Controller/1 -> WT_PWM/1
  Gain/1 -> LED_PWM/1
  Tip-Speed Ratio MPPT/2(V_WT) -> V_WT/1
  Lambda calculation/1(lambda) -> Sum/2

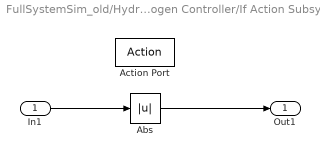
== system FullSystemSim_old/Hydrogen Controller/If Action Subsystem ==
  In1 : Inport
  Action Port : ActionPort  ActionPortLabel=else
  Abs : Abs
  Out1 : Outport
  wires:
  In1/1 -> Abs/1
  Abs/1 -> Out1/1

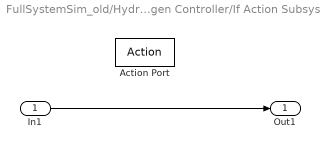
== system FullSystemSim_old/Hydrogen Controller/If Action Subsystem1 ==
  In1 : Inport
  Action Port : ActionPort  ActionPortLabel=if(u1 > 0)
  Out1 : Outport
  wires:
  In1/1 -> Out1/1

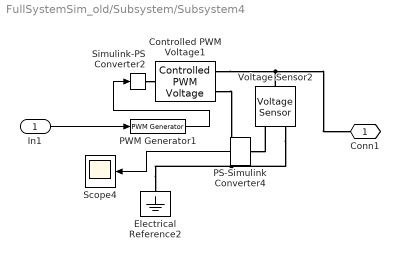
== system FullSystemSim_old/Subsystem/Subsystem4 ==
  In1 : Inport
  Controlled PWM Voltage1 : ee_lib/Integrated Circuits/Controlled PWM Voltage  F=490 Hz  TD=0 s  pulse_width_offset=0 s  pulse_min=0 s  Vmin=0 V  Vmax=5 V  Vm=5 V  pwm_or_av=1  event_type=1  sample_time=1e-6 s  u_min=0  u_max=1
      settings: InternalSimscapePortConfiguration="{\"Bottom\":[],\"Left\":[{\"id\":\"u\",\"label\":\"u\",\"type\":\"input\"}],\"Right\":[{\"id\":\"p2\",\"label\":\"PWM\",\"type\":\"foundation.electrical.electrical\"},{\"id\":\"n2\",\"label\":\"REF\",\"type\":\"foundation.electrical.electrical\"}],\"Top\":[]}"
  Electrical Reference2 : fl_lib/Electrical/Electrical Elements/Electrical Reference
  PS-Simulink Converter4 : nesl_utility/PS-Simulink Converter  PhysicalDomain=network_engine_domain  SubClassName=ps_output  LeftPortType=input  RightPortType=output  PseudoPeriodic=off  Frequencies=[]  Unit=inherit  AffineConversion=off
  PWM Generator1 : eePwmGenerator/PWM Generator  CarrCount=Up  Tper=0.001  Ts=5e-5
  Scope4 : Scope
  Simulink-PS Converter2 : nesl_utility/Simulink-PS Converter  PhysicalDomain=network_engine_domain  SubClassName=ps_input  LeftPortType=input  RightPortType=output  PseudoPeriodic=off  Frequencies=[]  NoiseDistribution=none  NoiseParameters=[]  Unit=1  AffineConversion=off  FilteringAndDerivatives=provide  SimscapeFilterOrder=1  InputFilterTimeConstant=0.001  UdotUserProvided=0
  Voltage Sensor2 : fl_lib/Electrical/Electrical Sensors/Voltage Sensor
  Conn1 : PMIOPort  Side=Right
  wires:
  In1/1 -> PWM Generator1/1
  PWM Generator1/1 -> Simulink-PS Converter2/1
  PS-Simulink Converter4/1 -> Scope4/1
  connections:
  PS-Simulink Converter4/LConn1 -- Voltage Sensor2/RConn1
  Electrical Reference2/LConn1 -- Controlled PWM Voltage1/RConn2 -- Voltage Sensor2/RConn2
  Controlled PWM Voltage1/RConn1 -- Conn1/RConn1 -- Voltage Sensor2/LConn1
  Simulink-PS Converter2/RConn1 -- Controlled PWM Voltage1/LConn1

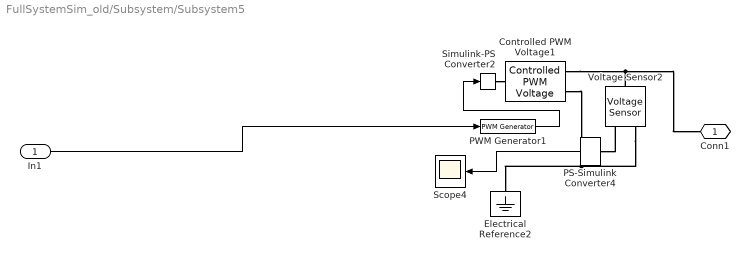
== system FullSystemSim_old/Subsystem/Subsystem5 ==
  In1 : Inport
  Controlled PWM Voltage1 : ee_lib/Integrated Circuits/Controlled PWM Voltage  F=490 Hz  TD=0 s  pulse_width_offset=0 s  pulse_min=0 s  Vmin=0 V  Vmax=5 V  Vm=5 V  pwm_or_av=1  event_type=1  sample_time=1e-6 s  u_min=0  u_max=1
      settings: InternalSimscapePortConfiguration="{\"Bottom\":[],\"Left\":[{\"id\":\"u\",\"label\":\"u\",\"type\":\"input\"}],\"Right\":[{\"id\":\"p2\",\"label\":\"PWM\",\"type\":\"foundation.electrical.electrical\"},{\"id\":\"n2\",\"label\":\"REF\",\"type\":\"foundation.electrical.electrical\"}],\"Top\":[]}"
  Electrical Reference2 : fl_lib/Electrical/Electrical Elements/Electrical Reference
  PS-Simulink Converter4 : nesl_utility/PS-Simulink Converter  PhysicalDomain=network_engine_domain  SubClassName=ps_output  LeftPortType=input  RightPortType=output  PseudoPeriodic=off  Frequencies=[]  Unit=inherit  AffineConversion=off
  PWM Generator1 : eePwmGenerator/PWM Generator  CarrCount=Up  Tper=0.001  Ts=5e-5
  Scope4 : Scope
  Simulink-PS Converter2 : nesl_utility/Simulink-PS Converter  PhysicalDomain=network_engine_domain  SubClassName=ps_input  LeftPortType=input  RightPortType=output  PseudoPeriodic=off  Frequencies=[]  NoiseDistribution=none  NoiseParameters=[]  Unit=1  AffineConversion=off  FilteringAndDerivatives=provide  SimscapeFilterOrder=1  InputFilterTimeConstant=0.001  UdotUserProvided=0
  Voltage Sensor2 : fl_lib/Electrical/Electrical Sensors/Voltage Sensor
  Conn1 : PMIOPort  Side=Right
  wires:
  In1/1 -> PWM Generator1/1
  PWM Generator1/1 -> Simulink-PS Converter2/1
  PS-Simulink Converter4/1 -> Scope4/1
  connections:
  PS-Simulink Converter4/LConn1 -- Voltage Sensor2/RConn1
  Voltage Sensor2/RConn2 -- Electrical Reference2/LConn1 -- Controlled PWM Voltage1/RConn2
  Voltage Sensor2/LConn1 -- Controlled PWM Voltage1/RConn1 -- Conn1/RConn1
  Simulink-PS Converter2/RConn1 -- Controlled PWM Voltage1/LConn1

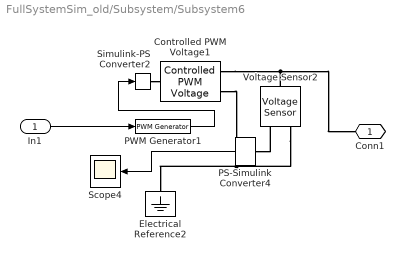
== system FullSystemSim_old/Subsystem/Subsystem6 ==
  In1 : Inport
  Controlled PWM Voltage1 : ee_lib/Integrated Circuits/Controlled PWM Voltage  F=490 Hz  TD=0 s  pulse_width_offset=0 s  pulse_min=0 s  Vmin=0 V  Vmax=5 V  Vm=5 V  pwm_or_av=1  event_type=1  sample_time=1e-6 s  u_min=0  u_max=1
      settings: InternalSimscapePortConfiguration="{\"Bottom\":[],\"Left\":[{\"id\":\"u\",\"label\":\"u\",\"type\":\"input\"}],\"Right\":[{\"id\":\"p2\",\"label\":\"PWM\",\"type\":\"foundation.electrical.electrical\"},{\"id\":\"n2\",\"label\":\"REF\",\"type\":\"foundation.electrical.electrical\"}],\"Top\":[]}"
  Electrical Reference2 : fl_lib/Electrical/Electrical Elements/Electrical Reference
  PS-Simulink Converter4 : nesl_utility/PS-Simulink Converter  PhysicalDomain=network_engine_domain  SubClassName=ps_output  LeftPortType=input  RightPortType=output  PseudoPeriodic=off  Frequencies=[]  Unit=inherit  AffineConversion=off
  PWM Generator1 : eePwmGenerator/PWM Generator  CarrCount=Up  Tper=0.001  Ts=5e-5
  Scope4 : Scope
  Simulink-PS Converter2 : nesl_utility/Simulink-PS Converter  PhysicalDomain=network_engine_domain  SubClassName=ps_input  LeftPortType=input  RightPortType=output  PseudoPeriodic=off  Frequencies=[]  NoiseDistribution=none  NoiseParameters=[]  Unit=1  AffineConversion=off  FilteringAndDerivatives=provide  SimscapeFilterOrder=1  InputFilterTimeConstant=0.001  UdotUserProvided=0
  Voltage Sensor2 : fl_lib/Electrical/Electrical Sensors/Voltage Sensor
  Conn1 : PMIOPort  Side=Right
  wires:
  In1/1 -> PWM Generator1/1
  PWM Generator1/1 -> Simulink-PS Converter2/1
  PS-Simulink Converter4/1 -> Scope4/1
  connections:
  PS-Simulink Converter4/LConn1 -- Voltage Sensor2/RConn1
  Voltage Sensor2/RConn2 -- Electrical Reference2/LConn1 -- Controlled PWM Voltage1/RConn2
  Voltage Sensor2/LConn1 -- Controlled PWM Voltage1/RConn1 -- Conn1/RConn1
  Simulink-PS Converter2/RConn1 -- Controlled PWM Voltage1/LConn1

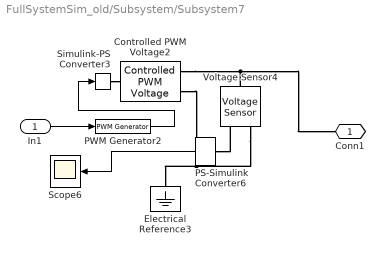
== system FullSystemSim_old/Subsystem/Subsystem7 ==
  In1 : Inport
  Controlled PWM Voltage2 : ee_lib/Integrated Circuits/Controlled PWM Voltage  F=490 Hz  TD=0 s  pulse_width_offset=0 s  pulse_min=0 s  Vmin=0 V  Vmax=5 V  Vm=5 V  pwm_or_av=1  event_type=1  sample_time=1e-6 s  u_min=0  u_max=1
      settings: InternalSimscapePortConfiguration="{\"Bottom\":[],\"Left\":[{\"id\":\"u\",\"label\":\"u\",\"type\":\"input\"}],\"Right\":[{\"id\":\"p2\",\"label\":\"PWM\",\"type\":\"foundation.electrical.electrical\"},{\"id\":\"n2\",\"label\":\"REF\",\"type\":\"foundation.electrical.electrical\"}],\"Top\":[]}"
  Electrical Reference3 : fl_lib/Electrical/Electrical Elements/Electrical Reference
  PS-Simulink Converter6 : nesl_utility/PS-Simulink Converter  PhysicalDomain=network_engine_domain  SubClassName=ps_output  LeftPortType=input  RightPortType=output  PseudoPeriodic=off  Frequencies=[]  Unit=inherit  AffineConversion=off
  PWM Generator2 : eePwmGenerator/PWM Generator  CarrCount=Up  Tper=0.001  Ts=5e-5
  Scope6 : Scope
  Simulink-PS Converter3 : nesl_utility/Simulink-PS Converter  PhysicalDomain=network_engine_domain  SubClassName=ps_input  LeftPortType=input  RightPortType=output  PseudoPeriodic=off  Frequencies=[]  NoiseDistribution=none  NoiseParameters=[]  Unit=1  AffineConversion=off  FilteringAndDerivatives=provide  SimscapeFilterOrder=1  InputFilterTimeConstant=0.001  UdotUserProvided=0
  Voltage Sensor4 : fl_lib/Electrical/Electrical Sensors/Voltage Sensor
  Conn1 : PMIOPort  Side=Right
  wires:
  PWM Generator2/1 -> Simulink-PS Converter3/1
  In1/1 -> PWM Generator2/1
  PS-Simulink Converter6/1 -> Scope6/1
  connections:
  Voltage Sensor4/LConn1 -- Controlled PWM Voltage2/RConn1 -- Conn1/RConn1
  Voltage Sensor4/RConn2 -- Electrical Reference3/LConn1 -- Controlled PWM Voltage2/RConn2
  PS-Simulink Converter6/LConn1 -- Voltage Sensor4/RConn1
  Simulink-PS Converter3/RConn1 -- Controlled PWM Voltage2/LConn1

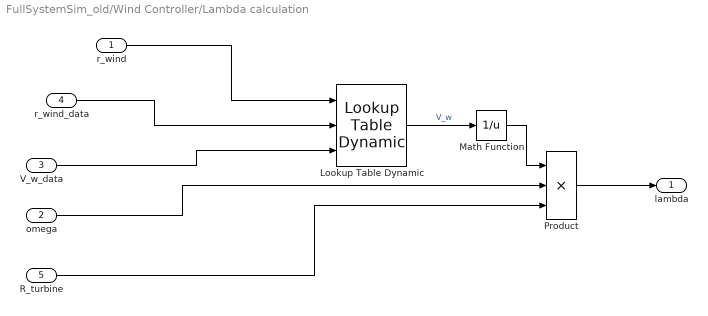
== system FullSystemSim_old/Wind Controller/Lambda calculation ==
  r_wind : Inport
  omega : Inport  Port=2
  V_w_data : Inport  Port=3
  r_wind_data : Inport  Port=4
  R_turbine : Inport  Port=5
  Lookup Table Dynamic : simulink/Lookup Tables/Lookup Table Dynamic  LookUpMeth=Interpolation-Use End Values  OutDataType=fixdt('double')  OutScaling=[]  OutputDataTypeScalingMode=Specify via dialog  OutDataTypeStr=double  DoSatur=off
  Math Function : Math  Operator=reciprocal  SignedPower=on  SaturateOnIntegerOverflow=on
  Product : Product  Inputs=3
  lambda : Outport
  wires:
  r_wind_data/1 -> Lookup Table Dynamic/2
  Product/1 -> lambda/1
  R_turbine/1 -> Product/3
  V_w_data/1 -> Lookup Table Dynamic/3
  Math Function/1 -> Product/1
  r_wind/1 -> Lookup Table Dynamic/1
  omega/1 -> Product/2
  Lookup Table Dynamic/1 -> Math Function/1  "V_w"

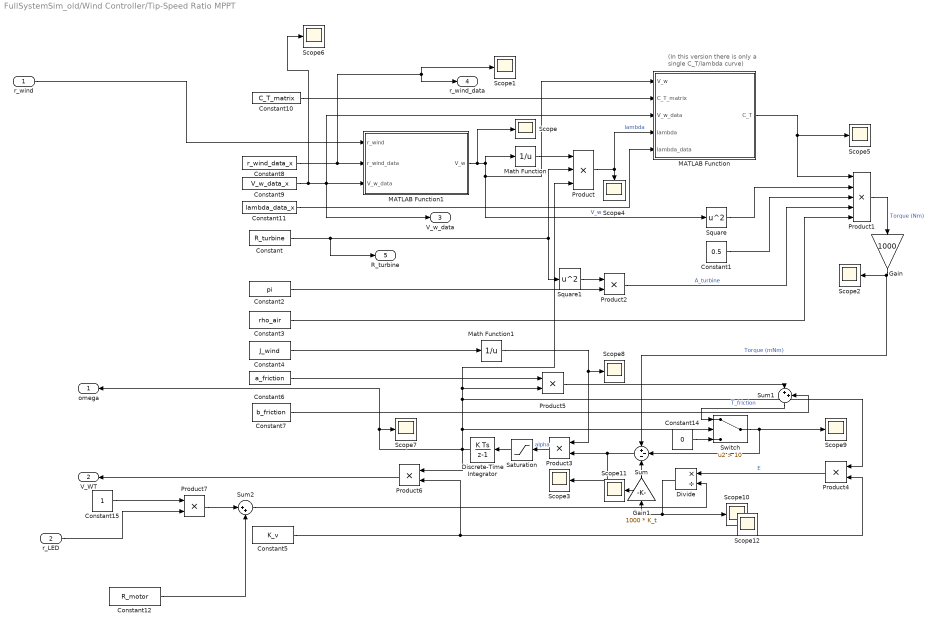
== system FullSystemSim_old/Wind Controller/Tip-Speed Ratio MPPT ==
  note: (In this version there is only
      | a single C_T/lambda curve)
  r_wind : Inport
  r_LED : Inport  Port=2
  Constant : Constant  Value=R_turbine
  Constant1 : Constant  Value=0.5
  Constant10 : Constant  Value=C_T_matrix
  Constant11 : Constant  Value=lambda_data_x
  Constant12 : Constant  Value=R_motor
  Constant14 : Constant  Value=0
  Constant15 : Constant
  Constant2 : Constant  Value=pi
  Constant3 : Constant  Value=rho_air
  Constant4 : Constant  Value=J_wind  SampleTime=step_size
  Constant5 : Constant  Value=K_v
  Constant6 : Constant  Value=a_friction
  Constant7 : Constant  Value=b_friction  SampleTime=step_size
  Constant8 : Constant  Value=r_wind_data_x
  Constant9 : Constant  Value=V_w_data_x
  Discrete-Time Integrator : DiscreteIntegrator  InitialCondition=omega_0  SampleTime=-1  ICPrevOutput=DiscIntNeverNeededParam  ICPrevScaledInput=DiscIntNeverNeededParam
  Divide : Product  Inputs=*/
  Gain : Gain  Gain=1000
  Gain1 : Gain  Gain=1000 * K_t
  MATLAB Function : MATLAB Function  TreatAsAtomicUnit=on
  MATLAB Function1 : MATLAB Function  TreatAsAtomicUnit=on
  Math Function : Math  Operator=reciprocal  SignedPower=on  SaturateOnIntegerOverflow=on
  Math Function1 : Math  Operator=reciprocal  SignedPower=on  SaturateOnIntegerOverflow=on
  Product : Product  Inputs=3
  Product1 : Product  Inputs=5
  Product{2..7} (6 alike) : Product
  Saturation : Saturate  UpperLimit=10000  LowerLimit=-40
  Scope{,1..12} (13 alike) : Scope
  Square : Math  Operator=square  SignedPower=on  SaturateOnIntegerOverflow=on
  Square1 : Math  Operator=square  SignedPower=on  SaturateOnIntegerOverflow=on
  Sum : Sum  Inputs=+--
  Sum1 : Sum  Inputs=|++
  Sum2 : Sum  Inputs=|++
  Switch : Switch  Criteria=u2 > Threshold  Threshold=10
  omega : Outport
  V_WT : Outport  Port=2
  V_w_data : Outport  Port=3
  r_wind_data : Outport  Port=4
  R_turbine : Outport  Port=5
  wires:
  Switch/1 -> Sum/2, Scope9/1
  Gain1/1 -> Sum/3, Scope11/1
  Product3/1 -> Saturation/1  "alpha"
  Math Function/1 -> Product/1
  Constant10/1 -> MATLAB Function/2(C_T_matrix)
  Product2/1 -> Product1/4  "A_turbine"
  Constant5/1 -> Product6/2, Product4/2
  Math Function1/1 -> Scope8/1, Product3/1
  Constant6/1 -> Product5/1
  Sum/1 -> Scope3/1, Product3/2
  Constant2/1 -> Product2/2
  Product4/1 -> Divide/1  "E"
  Divide/1 -> Gain1/1, Scope10/1
  Constant4/1 -> Math Function1/1
  Constant12/1 -> Sum2/2
  Square/1 -> Product1/2
  Constant3/1 -> Product1/5
  Constant7/1 -> Sum1/2
  r_wind/1 -> MATLAB Function1/1(r_wind)
  Product/1 -> MATLAB Function/4(lambda), Scope4/1  "lambda"
  Discrete-Time Integrator/1 -> Product/3, Product5/2, Product4/1, Switch/2, omega/1, Scope7/1, Product6/1
  Constant/1 -> R_turbine/1, Square1/1, Product/2
  Constant8/1 -> r_wind_data/1, Scope1/1, MATLAB Function1/2(r_wind_data)
  Constant9/1 -> Scope6/1, V_w_data/1, MATLAB Function/3(V_w_data), MATLAB Function1/3(V_w_data)
  Product6/1 -> V_WT/1
  Square1/1 -> Product2/1
  MATLAB Function/1(C_T) -> Product1/1, Scope5/1
  Gain/1 -> Sum/1, Scope2/1  "Torque (mNm)"
  Product7/1 -> Sum2/1
  r_LED/1 -> Product7/2
  Product5/1 -> Sum1/1
  Constant11/1 -> MATLAB Function/5(lambda_data)
  Constant14/1 -> Switch/3
  Saturation/1 -> Discrete-Time Integrator/1
  Sum2/1 -> Divide/2
  Constant1/1 -> Product1/3
  Sum1/1 -> Switch/1  "T_friction"
  Constant15/1 -> Product7/1
  Product1/1 -> Gain/1  "Torque (Nm)"
  MATLAB Function1/1(V_w) -> Math Function/1, Square/1, MATLAB Function/1(V_w), Scope/1  "V_w"

== matlab function FullSystemSim_old/Wind Controller/Tip-Speed Ratio MPPT/MATLAB Function1 ==
  data: r_wind input; V_w output; r_wind_data input; V_w_data input
function V_w = TableLookup(r_wind,r_wind_data,V_w_data)

V_w = interp1(r_wind_data,V_w_data,r_wind);

== matlab function FullSystemSim_old/Wind Controller/Tip-Speed Ratio MPPT/MATLAB Function ==
  data: V_w input; C_T output; C_T_matrix input; V_w_data input; lambda input; lambda_data input
function C_T = MatrixLookUp(V_w,C_T_matrix,V_w_data,lambda,lambda_data)
lambda = min( max(lambda, 0), 10);
C_T = interp1(lambda_data,interp1(V_w_data,C_T_matrix,V_w),lambda);
